simulink model "PM_Ser_DC_motors"  (R2022a)
settings: Solver=ode45  StartTime=0.0  StopTime=1  MaxStep=1e-3  RelTol=1e-4  AbsTol=1e-4  EnableMultiTasking=on
values from neighbouring files (symbols this model uses):
  Dm = 1e-4    (= 0.0001)    [dc_par.m]    (also in dcm_par.m = 6.04e-06)
  J = 1    [dc_par.m]    (also in dcm_par.m = 2.12e-06)
  Kv = 1.41e-2    (= 0.0141)    [dcm_par.m]
  Laf = 1.8    [dc_par.m]    (also in dcm_par.m = 0.0395)
  Ra = 0.6    [dc_par.m]    (also in dcm_par.m = 7)
  Ta = La/Ra    (= 0.02)    [dc_par.m]    (also in dcm_par.m = 0.0171428571429)
  Tm = 29    [dc_par.m]    (also in dcm_par.m = 0.00353)
  Va = 240    [dc_par.m]    (also in dcm_par.m = 6)
settings Model: Creator=Juri  LastModifiedBy=Juri
settings DataIOCC: LimitDataPoints=on  MaxDataPoints=10000  SaveFormat=Array  SignalLoggingSaveFormat=ModelDataLogs  SaveOutput=off  SaveState=on  ReturnWorkspaceOutputs=off  StateSaveName=x  TimeSaveName=t  SignalLoggingName=sigsOut
settings DebuggingCC: SaveWithParameterizedLinksMsg=none  UnderspecifiedInitializationDetection=Classic  MergeDetectMultiDrivingBlocksExec=none  SignalResolutionControl=TryResolveAllWithWarning  MultiTaskDSMMsg=warning  MultiTaskCondExecSysMsg=none  UnconnectedInputMsg=warning  UnconnectedOutputMsg=warning  UnconnectedLineMsg=warning
settings HardwareCC: ProdBitPerPointer=32  ProdBitPerSizeT=32  ProdBitPerPtrDiffT=32  ProdLargestAtomicFloat=None  ProdIntDivRoundTo=Undefined  ProdEndianess=Unspecified  ProdWordSize=32  ProdHWDeviceType=32-bit Generic  TargetUnknown=on
settings ModelReferenceCC: PropagateSignalLabelsOutOfModel=off
settings GRTTargetCC: CombineOutputUpdateFcns=off  GRTInterface=on
settings ConfigComp: CovMetricSettings=dw  CovSaveCumulativeToWorkspaceVar=on  CovSaveSingleToWorkspaceVar=on

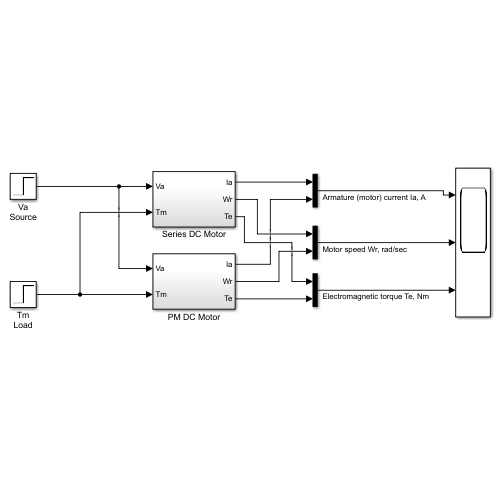
[thumbnail: Simulink's stored preview of the top-level diagram]
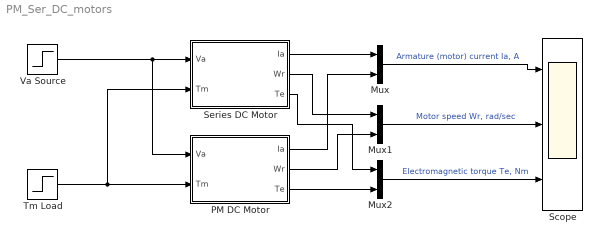
== system PM_Ser_DC_motors ==
  Mux : Mux  Inputs=2
  Mux1 : Mux  Inputs=2
  Mux2 : Mux  Inputs=2
  PM DC Motor : Subsystem
  Scope : Scope  NumInputPorts=3
  Series DC Motor : Subsystem
  Tm Load : Step  Time=0.5  After=Tm  SampleTime=0
  Va Source : Step  Time=0.05  After=Va  SampleTime=0
  wires:
  Va Source/1 -> Series DC Motor/1(Va), PM DC Motor/1(Va)
  Tm Load/1 -> Series DC Motor/2(Tm), PM DC Motor/2(Tm)
  Series DC Motor/1(Ia) -> Mux/1
  PM DC Motor/1(Ia) -> Mux/2
  Series DC Motor/2(Wr) -> Mux1/1
  PM DC Motor/2(Wr) -> Mux1/2
  Series DC Motor/3(Te) -> Mux2/1
  PM DC Motor/3(Te) -> Mux2/2
  Mux/1 -> Scope/1  "Armature (motor) current Ia, A"
  Mux1/1 -> Scope/2  "Motor speed Wr, rad/sec"
  Mux2/1 -> Scope/3  "Electromagnetic torque Te, Nm"

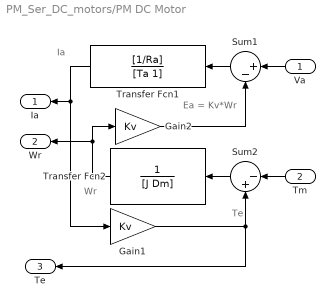
== system PM_Ser_DC_motors/PM DC Motor ==
  note: Ia
  note: Ea = Kv*Wr
  note: Wr
  note: Te
  Va : Inport
  Tm : Inport  Port=2
  Gain1 : Gain  Gain=Kv  SaturateOnIntegerOverflow=on  OutDataTypeStr=Inherit: Same as input  ParamDataTypeStr=Inherit: Same as input
  Gain2 : Gain  Gain=Kv  SaturateOnIntegerOverflow=on  OutDataTypeStr=Inherit: Same as input  ParamDataTypeStr=Inherit: Same as input
  Sum1 : Sum  Inputs=|+-  SaturateOnIntegerOverflow=on
  Sum2 : Sum  Inputs=|-+  SaturateOnIntegerOverflow=on
  Transfer Fcn1 : TransferFcn  Numerator=[1/Ra]  Denominator=[Ta 1]
  Transfer Fcn2 : TransferFcn  Denominator=[J Dm]
  Ia : Outport
  Wr : Outport  Port=2
  Te : Outport  Port=3
  wires:
  Sum1/1 -> Transfer Fcn1/1
  Gain2/1 -> Sum1/2
  Sum2/1 -> Transfer Fcn2/1
  Transfer Fcn1/1 -> Gain1/1, Ia/1
  Gain1/1 -> Te/1, Sum2/2
  Va/1 -> Sum1/1
  Tm/1 -> Sum2/1
  Transfer Fcn2/1 -> Gain2/1, Wr/1

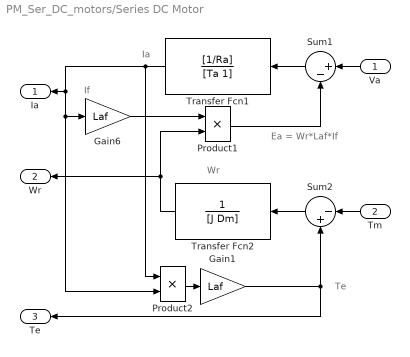
== system PM_Ser_DC_motors/Series DC Motor ==
  note: Ia
  note: If
  note: Ea = Wr*Laf*If
  note: Wr
  note: Te
  Va : Inport
  Tm : Inport  Port=2
  Gain1 : Gain  Gain=Laf  SaturateOnIntegerOverflow=on  OutDataTypeStr=Inherit: Same as input  ParamDataTypeStr=Inherit: Same as input
  Gain6 : Gain  Gain=Laf  SaturateOnIntegerOverflow=on  OutDataTypeStr=Inherit: Same as input  ParamDataTypeStr=Inherit: Same as input
  Product1 : Product  SaturateOnIntegerOverflow=on  OutDataTypeStr=Inherit: Same as first input
  Product2 : Product  SaturateOnIntegerOverflow=on  OutDataTypeStr=Inherit: Same as first input
  Sum1 : Sum  Inputs=|+-  SaturateOnIntegerOverflow=on
  Sum2 : Sum  Inputs=|-+  SaturateOnIntegerOverflow=on
  Transfer Fcn1 : TransferFcn  Numerator=[1/Ra]  Denominator=[Ta 1]
  Transfer Fcn2 : TransferFcn  Denominator=[J Dm]
  Ia : Outport
  Wr : Outport  Port=2
  Te : Outport  Port=3
  wires:
  Gain6/1 -> Product1/1
  Sum1/1 -> Transfer Fcn1/1
  Transfer Fcn2/1 -> Product1/2, Wr/1
  Product1/1 -> Sum1/2
  Sum2/1 -> Transfer Fcn2/1
  Product2/1 -> Gain1/1
  Transfer Fcn1/1 -> Product2/1, Gain6/1, Product2/2, Ia/1
  Gain1/1 -> Sum2/2, Te/1
  Va/1 -> Sum1/1
  Tm/1 -> Sum2/1
